simulink model "parkingNavigationTest"  (R2021b)
settings: Solver=VariableStepAuto  StartTime=0.0  StopTime=3600  FixedStep=0.01  RelTol=1e-3
model workspace (MAT data in the model file):
  enableTransmit = 1
libraries: matrix_library x10, sharedutil x4, simulink x3, aerolibutil x2
(part 2 of 2)

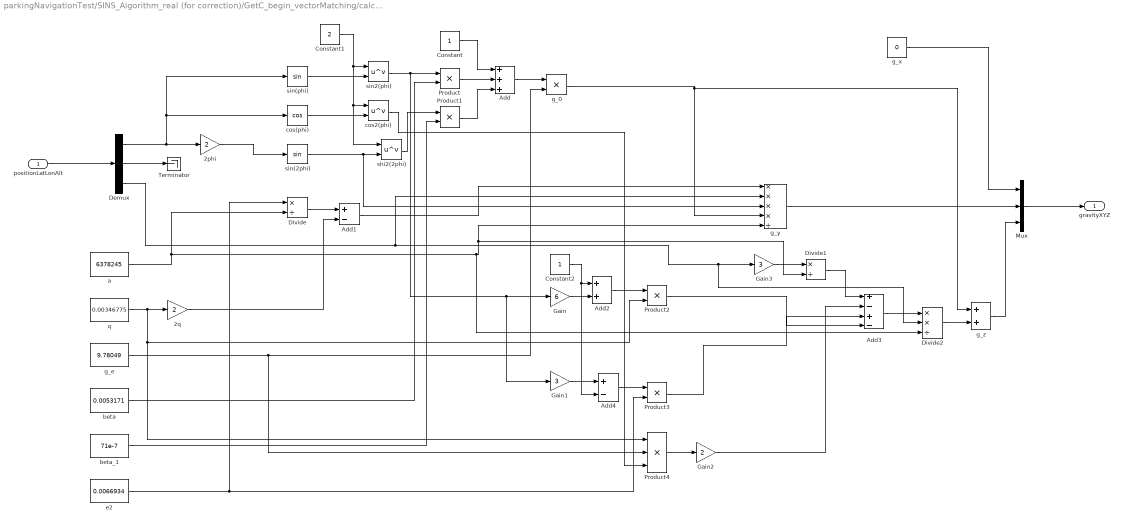
== system parkingNavigationTest/SINS_Algorithm_real (for correction)/GetC_begin_vectorMatching/calculate_GravityXYZ ==
  positionLatLonAlt : Inport
  2phi : Gain  Gain=2
  2q : Gain  Gain=2
  Add : Sum  Inputs=+++
  Add1 : Sum  Inputs=+-
  Add2 : Sum
  Add3 : Sum  Inputs=+-+-
  Add4 : Sum  Inputs=+-
  Constant : Constant
  Constant1 : Constant  Value=2
  Constant2 : Constant
  Demux : Demux  Outputs=3
  Divide : Product  Inputs=*/
  Divide1 : Product  Inputs=*/
  Divide2 : Product  Inputs=**/
  Gain : Gain  Gain=6
  Gain1 : Gain  Gain=3
  Gain2 : Gain  Gain=2
  Gain3 : Gain  Gain=3
  Mux : Mux  Inputs=3
  Product{,1..3} (4 alike) : Product
  Product4 : Product  Inputs=3
  Terminator : Terminator
  a : Constant  Value=6378245
  beta : Constant  Value=0.0053171
  beta_1 : Constant  Value=71e-7
  cos(phi) : Trigonometry  Operator=cos
  cos2(phi) : Math  Operator=pow  SaturateOnIntegerOverflow=on
  e2 : Constant  Value=0.0066934
  g_0 : Product
  g_e : Constant  Value=9.78049
  g_x : Constant  Value=0
  g_y : Product  Inputs=****/
  g_z : Sum
  q : Constant  Value=0.00346775
  shi2(2phi) : Math  Operator=pow  SaturateOnIntegerOverflow=on
  sin(2phi) : Trigonometry
  sin(phi) : Trigonometry
  sin2(phi) : Math  Operator=pow  SaturateOnIntegerOverflow=on
  gravityXYZ : Outport
  wires:
  positionLatLonAlt/1 -> Demux/1
  Demux/2 -> Terminator/1
  Mux/1 -> gravityXYZ/1
  Demux/1 -> cos(phi)/1, sin(phi)/1, 2phi/1
  2phi/1 -> sin(2phi)/1
  sin(phi)/1 -> sin2(phi)/2
  Constant1/1 -> cos2(phi)/1, shi2(2phi)/1, sin2(phi)/1
  sin(2phi)/1 -> g_y/3, shi2(2phi)/2
  beta/1 -> Product/2
  sin2(phi)/1 -> Gain1/1, Gain/1, Product/1
  shi2(2phi)/1 -> Product1/1
  beta_1/1 -> Product1/2
  Product/1 -> Add/2
  Constant/1 -> Add/1
  Product1/1 -> Add/3
  Add/1 -> g_0/1
  g_e/1 -> Product4/2, g_0/2
  e2/1 -> Product3/2, Divide/1
  a/1 -> Divide2/3, Divide1/2, g_y/5, Divide/2
  Divide/1 -> Add1/1
  q/1 -> Product4/1, Product2/2, 2q/1
  2q/1 -> Add1/2
  Add1/1 -> g_y/1
  Demux/3 -> g_y/2, Divide2/2, Gain3/1
  g_0/1 -> g_z/1, g_y/4
  g_y/1 -> Mux/2
  cos(phi)/1 -> cos2(phi)/2
  Gain/1 -> Add2/2
  Constant2/1 -> Add4/2, Add2/1
  Add2/1 -> Product2/1
  Product2/1 -> Add3/4
  Gain1/1 -> Add4/1
  Add4/1 -> Product3/1
  Product3/1 -> Add3/3
  Product4/1 -> Gain2/1
  cos2(phi)/1 -> Product4/3
  Gain2/1 -> Add3/2
  Gain3/1 -> Divide1/1
  Divide1/1 -> Add3/1
  Add3/1 -> Divide2/1
  Divide2/1 -> g_z/2
  g_z/1 -> Mux/3
  g_x/1 -> Mux/1

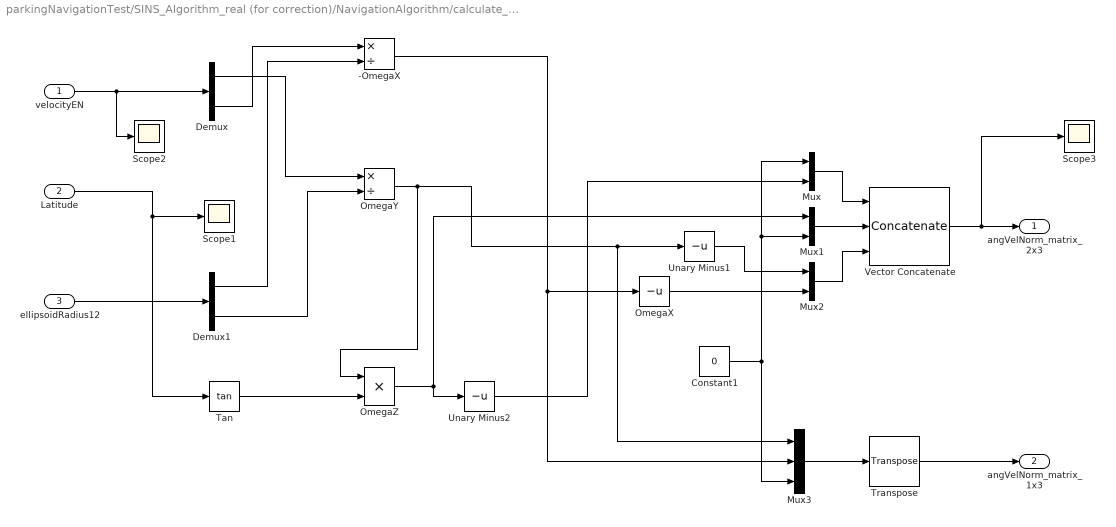
== system parkingNavigationTest/SINS_Algorithm_real (for correction)/NavigationAlgorithm/calculate_AngVelNorm_matrix ==
  velocityEN : Inport
  Latitude : Inport  Port=2
  ellipsoidRadius12 : Inport  Port=3
  -OmegaX : Product  Inputs=*/
  Constant1 : Constant  Value=0
  Demux : Demux  Outputs=2
  Demux1 : Demux  Outputs=2
  Mux : Mux  Inputs=2
  Mux1 : Mux  Inputs=2
  Mux2 : Mux  Inputs=2
  Mux3 : Mux  Inputs=3
  OmegaX : UnaryMinus
  OmegaY : Product  Inputs=*/
  OmegaZ : Product  Inputs=**
  Scope1 : Scope
  Scope2 : Scope
  Scope3 : Scope
  Tan : Trigonometry  Operator=tan
  Transpose : matrix_library/Transpose
      settings: SourceProductBaseCode=SL
  Unary Minus1 : UnaryMinus
  Unary Minus2 : UnaryMinus
  Vector Concatenate : Concatenate  NumInputs=3  Mode=Multidimensional array  ConcatenateDimension=2
  angVelNorm_matrix_2x3 : Outport
  angVelNorm_matrix_1x3 : Outport  Port=2
  wires:
  velocityEN/1 -> Scope2/1, Demux/1
  ellipsoidRadius12/1 -> Demux1/1
  Demux/2 -> -OmegaX/1
  Demux1/1 -> -OmegaX/2
  -OmegaX/1 -> Mux3/2, OmegaX/1
  OmegaX/1 -> Mux2/2
  Demux/1 -> OmegaY/1
  Demux1/2 -> OmegaY/2
  OmegaY/1 -> OmegaZ/1, Mux3/1, Unary Minus1/1
  Unary Minus1/1 -> Mux2/1
  Tan/1 -> OmegaZ/2
  Latitude/1 -> Scope1/1, Tan/1
  OmegaZ/1 -> Unary Minus2/1, Mux1/1
  Unary Minus2/1 -> Mux/2
  Constant1/1 -> Mux3/3, Mux/1, Mux1/2
  Mux1/1 -> Vector Concatenate/2
  Mux/1 -> Vector Concatenate/1
  Mux2/1 -> Vector Concatenate/3
  Vector Concatenate/1 -> Scope3/1, angVelNorm_matrix_2x3/1
  Mux3/1 -> Transpose/1
  Transpose/1 -> angVelNorm_matrix_1x3/1

== system parkingNavigationTest/SINS_Algorithm_real (for correction)/NavigationAlgorithm/calculate_AngVelNorm_matrix_3CH ==
  velocityENH : Inport
  Latitude : Inport  Port=2
  ellipsoidRadius12 : Inport  Port=3
  Constant : Constant  Value=0
  Create 3x3 Matrix : sharedutil/Create 3x3 Matrix  aMode=aMode
      settings: SourceProductBaseCode=AE,PW,DR,MT,UV,VE
  Demux : Demux  Outputs=3
  Demux1 : Demux  Outputs=2
  Divide : Product  Inputs=*/
  OmegaX : UnaryMinus
  OmegaY : Product  Inputs=*/
  OmegaZ : Product  Inputs=**/
  Tan : Trigonometry  Operator=tan
  Terminator : Terminator
  Unary Minus1 : UnaryMinus
  Unary Minus2 : UnaryMinus
  angVelNorm_matrix : Outport
  wires:
  velocityENH/1 -> Demux/1
  ellipsoidRadius12/1 -> Demux1/1
  Demux/2 -> Divide/1
  Demux1/1 -> Divide/2
  Divide/1 -> Create 3x3 Matrix/8, OmegaX/1
  OmegaX/1 -> Create 3x3 Matrix/6
  Demux/1 -> OmegaZ/1, OmegaY/1
  Demux1/2 -> OmegaZ/3, OmegaY/2
  OmegaY/1 -> Unary Minus1/1, Create 3x3 Matrix/7
  Unary Minus1/1 -> Create 3x3 Matrix/3
  Tan/1 -> OmegaZ/2
  Latitude/1 -> Tan/1
  OmegaZ/1 -> Unary Minus2/1, Create 3x3 Matrix/2
  Unary Minus2/1 -> Create 3x3 Matrix/4
  Constant/1 -> Create 3x3 Matrix/9, Create 3x3 Matrix/5, Create 3x3 Matrix/1
  Create 3x3 Matrix/1 -> angVelNorm_matrix/1
  Demux/3 -> Terminator/1

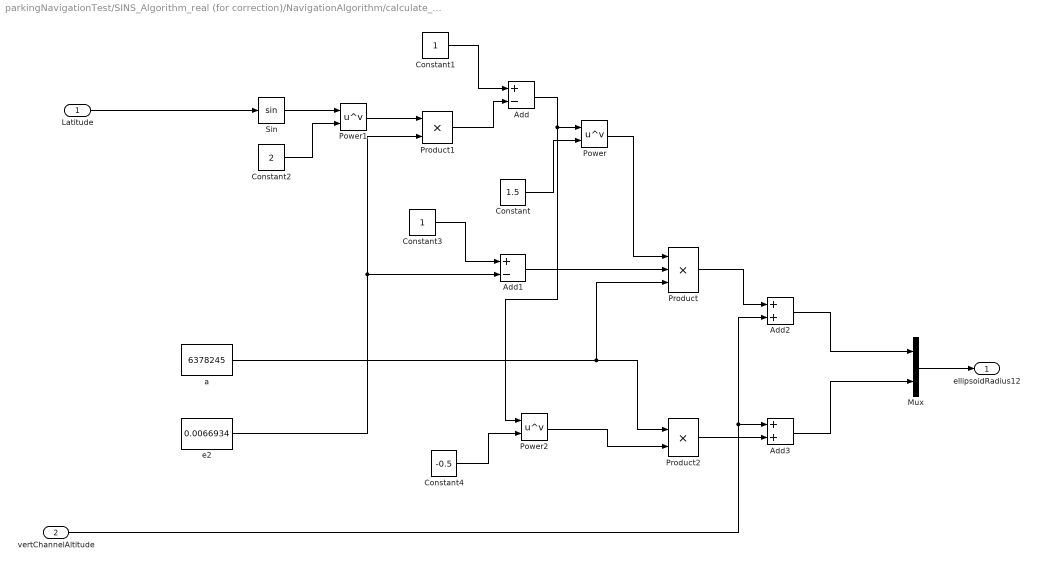
== system parkingNavigationTest/SINS_Algorithm_real (for correction)/NavigationAlgorithm/calculate_EllipsoidRadius12 ==
  Latitude : Inport
  vertChannelAltitude : Inport  Port=2
  Add : Sum  Inputs=+-
  Add1 : Sum  Inputs=+-
  Add2 : Sum
  Add3 : Sum
  Constant : Constant  Value=1.5
  Constant1 : Constant
  Constant2 : Constant  Value=2
  Constant3 : Constant
  Constant4 : Constant  Value=-0.5
  Mux : Mux  Inputs=2
  Power : Math  Operator=pow  SaturateOnIntegerOverflow=on
  Power1 : Math  Operator=pow  SaturateOnIntegerOverflow=on
  Power2 : Math  Operator=pow  SaturateOnIntegerOverflow=on
  Product : Product  Inputs=3
  Product1 : Product
  Product2 : Product
  Sin : Trigonometry
  a : Constant  Value=6378245
  e2 : Constant  Value=0.0066934
  ellipsoidRadius12 : Outport
  wires:
  Mux/1 -> ellipsoidRadius12/1
  Constant1/1 -> Add/1
  Product1/1 -> Add/2
  Power1/1 -> Product1/1
  Sin/1 -> Power1/1
  Constant2/1 -> Power1/2
  Latitude/1 -> Sin/1
  e2/1 -> Add1/2, Product1/2
  Add/1 -> Power2/1, Power/1
  Constant/1 -> Power/2
  Power/1 -> Product/1
  Constant3/1 -> Add1/1
  Add1/1 -> Product/2
  a/1 -> Product2/1, Product/3
  Product/1 -> Add2/1
  vertChannelAltitude/1 -> Add2/2, Add3/1
  Add2/1 -> Mux/1
  Constant4/1 -> Power2/2
  Power2/1 -> Product2/2
  Product2/1 -> Add3/2
  Add3/1 -> Mux/2

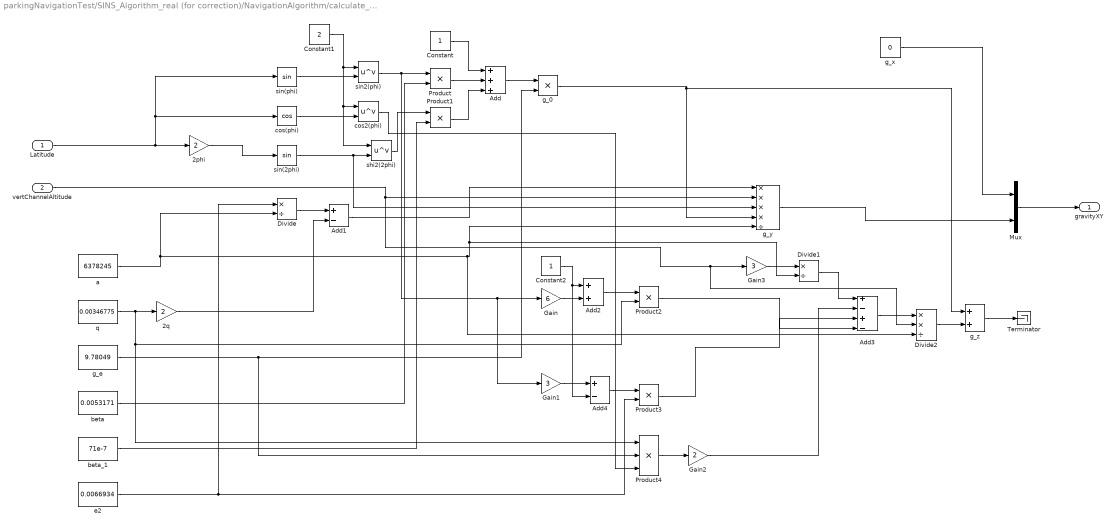
== system parkingNavigationTest/SINS_Algorithm_real (for correction)/NavigationAlgorithm/calculate_GravityXY ==
  Latitude : Inport
  vertChannelAltitude : Inport  Port=2
  2phi : Gain  Gain=2
  2q : Gain  Gain=2
  Add : Sum  Inputs=+++
  Add1 : Sum  Inputs=+-
  Add2 : Sum
  Add3 : Sum  Inputs=+-+-
  Add4 : Sum  Inputs=+-
  Constant : Constant
  Constant1 : Constant  Value=2
  Constant2 : Constant
  Divide : Product  Inputs=*/
  Divide1 : Product  Inputs=*/
  Divide2 : Product  Inputs=**/
  Gain : Gain  Gain=6
  Gain1 : Gain  Gain=3
  Gain2 : Gain  Gain=2
  Gain3 : Gain  Gain=3
  Mux : Mux  Inputs=2
  Product{,1..3} (4 alike) : Product
  Product4 : Product  Inputs=3
  Terminator : Terminator
  a : Constant  Value=6378245
  beta : Constant  Value=0.0053171
  beta_1 : Constant  Value=71e-7
  cos(phi) : Trigonometry  Operator=cos
  cos2(phi) : Math  Operator=pow  SaturateOnIntegerOverflow=on
  e2 : Constant  Value=0.0066934
  g_0 : Product
  g_e : Constant  Value=9.78049
  g_x : Constant  Value=0
  g_y : Product  Inputs=****/
  g_z : Sum
  q : Constant  Value=0.00346775
  shi2(2phi) : Math  Operator=pow  SaturateOnIntegerOverflow=on
  sin(2phi) : Trigonometry
  sin(phi) : Trigonometry
  sin2(phi) : Math  Operator=pow  SaturateOnIntegerOverflow=on
  gravityXY : Outport
  wires:
  Mux/1 -> gravityXY/1
  Latitude/1 -> cos(phi)/1, sin(phi)/1, 2phi/1
  2phi/1 -> sin(2phi)/1
  sin(phi)/1 -> sin2(phi)/2
  Constant1/1 -> cos2(phi)/1, shi2(2phi)/1, sin2(phi)/1
  sin(2phi)/1 -> g_y/3, shi2(2phi)/2
  beta/1 -> Product/2
  sin2(phi)/1 -> Gain1/1, Gain/1, Product/1
  shi2(2phi)/1 -> Product1/1
  beta_1/1 -> Product1/2
  Product/1 -> Add/2
  Constant/1 -> Add/1
  Product1/1 -> Add/3
  Add/1 -> g_0/1
  g_e/1 -> Product4/2, g_0/2
  e2/1 -> Product3/2, Divide/1
  a/1 -> Divide2/3, Divide1/2, g_y/5, Divide/2
  Divide/1 -> Add1/1
  q/1 -> Product4/1, Product2/2, 2q/1
  2q/1 -> Add1/2
  Add1/1 -> g_y/1
  vertChannelAltitude/1 -> Divide2/2, Gain3/1, g_y/2
  g_0/1 -> g_z/1, g_y/4
  g_y/1 -> Mux/2
  cos(phi)/1 -> cos2(phi)/2
  Gain/1 -> Add2/2
  Constant2/1 -> Add4/2, Add2/1
  Add2/1 -> Product2/1
  Product2/1 -> Add3/4
  Gain1/1 -> Add4/1
  Add4/1 -> Product3/1
  Product3/1 -> Add3/3
  Product4/1 -> Gain2/1
  cos2(phi)/1 -> Product4/3
  Gain2/1 -> Add3/2
  Gain3/1 -> Divide1/1
  Divide1/1 -> Add3/1
  Add3/1 -> Divide2/1
  Divide2/1 -> g_z/2
  g_z/1 -> Terminator/1
  g_x/1 -> Mux/1

== system parkingNavigationTest/SINS_Algorithm_real (for correction)/NavigationAlgorithm/calculate_U_matrix ==
  U_earth : Inport
  Latitude : Inport  Port=2
  Constant : Constant  Value=0
  Cos : Trigonometry  Operator=cos
  Mux : Mux  Inputs=2
  Mux1 : Mux  Inputs=2
  Mux2 : Mux  Inputs=2
  Mux3 : Mux  Inputs=3
  Sin : Trigonometry
  Transpose : matrix_library/Transpose
      settings: SourceProductBaseCode=SL
  U_y : Product
  U_z : Product
  Unary Minus : UnaryMinus
  Unary Minus1 : UnaryMinus
  Vector Concatenate : Concatenate  NumInputs=3  Mode=Multidimensional array  ConcatenateDimension=2
  U_matrix_2x3 : Outport
  U_matrix_1x3 : Outport  Port=2
  wires:
  Latitude/1 -> Sin/1, Cos/1
  U_earth/1 -> U_z/1, U_y/1
  Cos/1 -> U_y/2
  U_y/1 -> Mux3/1, Unary Minus/1
  Unary Minus/1 -> Mux2/1
  Sin/1 -> U_z/2
  U_z/1 -> Mux1/1, Unary Minus1/1
  Unary Minus1/1 -> Mux/2
  Mux/1 -> Vector Concatenate/1
  Mux2/1 -> Vector Concatenate/3
  Mux1/1 -> Vector Concatenate/2
  Constant/1 -> Mux3/3, Mux3/2, Mux/1, Mux1/2, Mux2/2
  Vector Concatenate/1 -> U_matrix_2x3/1
  Mux3/1 -> Transpose/1
  Transpose/1 -> U_matrix_1x3/1

== system parkingNavigationTest/SINS_Algorithm_real (for correction)/NavigationAlgorithm/calculate_U_matrix_3CH ==
  U_earth : Inport
  Latitude : Inport  Port=2
  Constant : Constant  Value=0
  Cos : Trigonometry  Operator=cos
  Create 3x3 Matrix : sharedutil/Create 3x3 Matrix  aMode=aMode
      settings: SourceProductBaseCode=AE,PW,DR,MT,UV,VE
  Product : Product
  Product1 : Product
  Sin : Trigonometry
  Unary Minus : UnaryMinus
  Unary Minus1 : UnaryMinus
  U_matrix : Outport
  wires:
  Latitude/1 -> Sin/1, Cos/1
  U_earth/1 -> Product1/1, Product/1
  Cos/1 -> Product/2
  Product/1 -> Unary Minus/1, Create 3x3 Matrix/7
  Unary Minus/1 -> Create 3x3 Matrix/3
  Sin/1 -> Product1/2
  Product1/1 -> Unary Minus1/1, Create 3x3 Matrix/2
  Unary Minus1/1 -> Create 3x3 Matrix/4
  Constant/1 -> Create 3x3 Matrix/9, Create 3x3 Matrix/8, Create 3x3 Matrix/6, Create 3x3 Matrix/5, Create 3x3 Matrix/1
  Create 3x3 Matrix/1 -> U_matrix/1

== system parkingNavigationTest/SINS_Algorithm_real (for correction)/NavigationAlgorithm/eraseAccelZ ==
  accelerationXYZ : Inport
  Demux : Demux  Outputs=3
  Mux : Mux  Inputs=2
  Terminator : Terminator
  accelerationXY : Outport
  wires:
  accelerationXYZ/1 -> Demux/1
  Demux/1 -> Mux/1
  Demux/2 -> Mux/2
  Mux/1 -> accelerationXY/1
  Demux/3 -> Terminator/1

== system parkingNavigationTest/SINS_Algorithm_real (for correction)/OrientationAlgorithm/C to Orientation Angles ==
  C : Inport
  "C(1, 1)" : Selector  NumberOfDimensions=2  InputPortWidth=3  IndexOptions=Index vector (dialog),Index vector (dialog)  Indices=1,1  OutputSizes=1,1
  "C(2, 1)" : Selector  NumberOfDimensions=2  InputPortWidth=3  IndexOptions=Index vector (dialog),Index vector (dialog)  Indices=2,1  OutputSizes=1,1
  "C(2, 2)" : Selector  NumberOfDimensions=2  InputPortWidth=3  IndexOptions=Index vector (dialog),Index vector (dialog)  Indices=2,2  OutputSizes=1,1
  "C(2, 3)" : Selector  NumberOfDimensions=2  InputPortWidth=3  IndexOptions=Index vector (dialog),Index vector (dialog)  Indices=2,3  OutputSizes=1,1
  "C(3, 1)" : Selector  NumberOfDimensions=2  InputPortWidth=3  IndexOptions=Index vector (dialog),Index vector (dialog)  Indices=3,1  OutputSizes=1,1
  Divide2 : Product  Inputs=*/
  Divide3 : Product  Inputs=*/
  Mux : Mux  Inputs=3
  Sin3 : Trigonometry  Operator=atan
  Sin4 : Trigonometry  Operator=atan
  Sin5 : Trigonometry  Operator=asin
  Unary Minus : UnaryMinus
  Unary Minus3 : UnaryMinus
  RollPitchYaw : Outport
  wires:
  Divide2/1 -> Sin3/1
  "C(2, 2)"/1 -> Divide2/2
  Divide3/1 -> Sin4/1
  "C(3, 1)"/1 -> Unary Minus3/1
  Sin3/1 -> Mux/1
  Mux/1 -> RollPitchYaw/1
  C/1 -> "C(2, 3)"/1, "C(2, 2)"/1, "C(2, 1)"/1, "C(3, 1)"/1, "C(1, 1)"/1
  "C(1, 1)"/1 -> Divide3/2
  "C(2, 1)"/1 -> Sin5/1
  Unary Minus3/1 -> Divide3/1
  "C(2, 3)"/1 -> Unary Minus/1
  Unary Minus/1 -> Divide2/1
  Sin5/1 -> Mux/2
  Sin4/1 -> Mux/3

== system parkingNavigationTest/SINS_Algorithm_real (for correction)/OrientationAlgorithm/Skew symmetric matrix  ==
  angVel_x : Inport
  angVel_y : Inport  Port=2
  angVel_z : Inport  Port=3
  Constant5 : Constant  Value=0
  Mux1 : Mux  Inputs=3
  Mux2 : Mux  Inputs=3
  Mux3 : Mux  Inputs=3
  Unary Minus1 : UnaryMinus
  Unary Minus2 : UnaryMinus
  Unary Minus6 : UnaryMinus
  get angVel_matrix : Concatenate  NumInputs=3  Mode=Multidimensional array  ConcatenateDimension=2
  angVel_matrix : Outport
  wires:
  Mux3/1 -> get angVel_matrix/3
  Unary Minus1/1 -> Mux3/2
  Unary Minus2/1 -> Mux1/3
  angVel_x/1 -> Mux2/3, Unary Minus1/1
  get angVel_matrix/1 -> angVel_matrix/1
  Constant5/1 -> Mux3/3, Mux2/2, Mux1/1
  Mux1/1 -> get angVel_matrix/1
  Mux2/1 -> get angVel_matrix/2
  angVel_y/1 -> Unary Minus2/1, Mux3/1
  Unary Minus6/1 -> Mux2/1
  angVel_z/1 -> Unary Minus6/1, Mux1/2

== matlab function parkingNavigationTest/SINS_Algorithm_real (for correction)/GetC_begin_easy/calculate C_begin ==
  data: u input; y output
function y = fcn(u)

y1 = [ u(5) * u(6); 
    u(2); 
    -u(5) * u(3) ];
y2 = [ -u(4) * u(6) * u(2) + u(1) * u(3); 
    u(4) * u(5); 
    u(4) * u(3) * u(2) + u(1) * u(6) ];
y3 = [ u(1) * u(6) * u(2) + u(4) * u(3);
    -u(1) * u(5);
    -u(1) * u(3) * u(2) + u(4) * u(6)];
y = [ y1 y2 y3 ];

== matlab function parkingNavigationTest/SINS_Algorithm_ideal/GetC_begin_easy/calculate C_begin ==
  data: u input; y output
function y = fcn(u)

y1 = [ u(5) * u(6); 
    u(2); 
    -u(5) * u(3) ];
y2 = [ -u(4) * u(6) * u(2) + u(1) * u(3); 
    u(4) * u(5); 
    u(4) * u(3) * u(2) + u(1) * u(6) ];
y3 = [ u(1) * u(6) * u(2) + u(4) * u(3);
    -u(1) * u(5);
    -u(1) * u(3) * u(2) + u(4) * u(6)];
y = [ y1 y2 y3 ];
